simulink model "DC_motor_disc"  (R2022b)
settings: Solver=VariableStepAuto  StartTime=0.0  StopTime=1  RelTol=1e-7
PreLoadFcn:
  | P = eye(2);
  | Q_prev = [0.5 0; 0 0.5];
  | R_prev = eye(2);
PostLoadFcn:
  | P = eye(2);
  | Q_prev = [0.5 0; 0 0.5];
  | R_prev = eye(2);
InitFcn:
  | P = eye(2);
  | Q_prev = [0.5 0; 0 0.5];
  | R_prev = eye(2);
StartFcn:
  | P = eye(2);
  | Q_prev = [0.5 0; 0 0.5];
  | R_prev = eye(2);
values from neighbouring files (symbols this model uses):
  g = 9.81    [DC_motor_params.m]
  l = 0.05    [DC_motor_params.m]
  m = 5    [DC_motor_params.m]
  Ts = 10^-5    (= 1e-05)    [DC_motor_params.m]
undefined symbols (not defined in the file or in its folder): DiscIntNeverNeededParam, sigbuilder_block
libraries: simulink x3, spsControlledVoltageSourceLib x1, spsCurrentMeasurementLib x1, spsDCMachineLib x1, spsDCVoltageSourceLib x1, slpidlib x1, spsVoltageMeasurementLib x1, spspowerguiLib x1
settings Model: Creator=Pascal  LastModifiedBy=Pascal
settings DataIOCC: ReturnWorkspaceOutputs=off
settings DebuggingCC: AlgebraicLoopMsg=none
settings ModelReferenceCC: ModelReferenceMinAlgLoopOccurrences=on

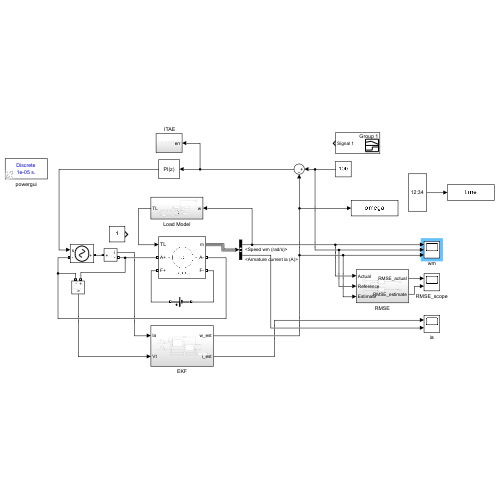
[thumbnail: Simulink's stored preview of the top-level diagram]
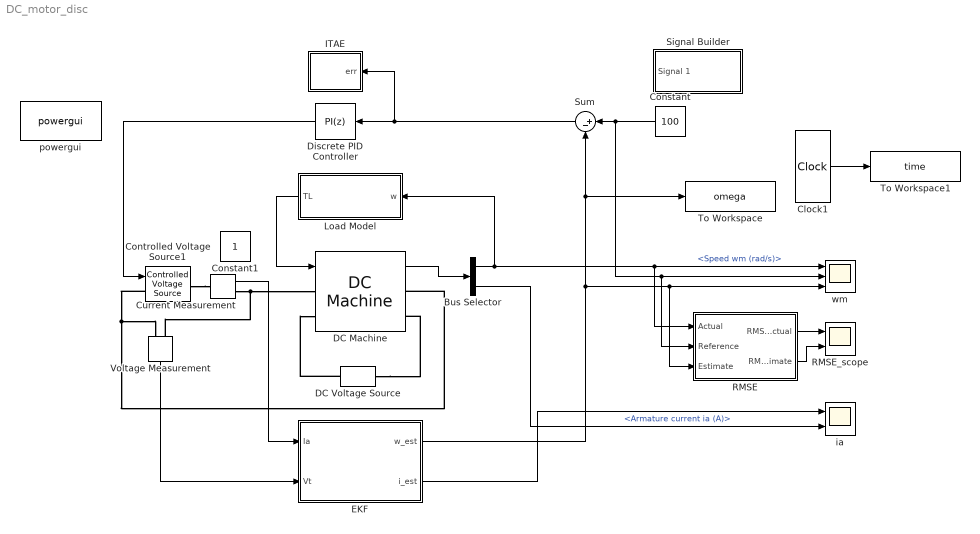
== system DC_motor_disc ==
  " ITAE" : Subsystem
  Bus Selector : BusSelector  OutputSignals=Speed wm (rad/s),Armature current ia (A)
  Clock1 : DigitalClock  SampleTime=Ts
  Constant : Constant  Value=100  SampleTime=Ts
  Constant1 : Constant
  Controlled Voltage Source1 : spsControlledVoltageSourceLib/Controlled Voltage Source  Initialize=off  Source_Type=DC  Amplitude=0  Phase=0  Frequency=0  Measurements=Voltage
  Current Measurement : spsCurrentMeasurementLib/Current Measurement  PhasorSimulation=off  OutputType=Complex  PSBequivalent=0
  DC Machine : spsDCMachineLib/DC Machine  PresetModel=No  MechanicalLoad=Torque TL  FieldType=Wound  ShowDetailedParameters=on  MeasurementBus=off  RLa=[2.581 0.028]  RLf=[240 120]  Laf=0.9483  MachineConstant=Torque constant (N.m/A)  Ke=1.8  Kt=1.8  J=0.02215  Bm=0.002953  Tf=0.5161  w0=0  Ifinit=1.25  TsPowergui=0  TsBlock=Ts
  DC Voltage Source : spsDCVoltageSourceLib/DC Voltage Source  Amplitude=300  Measurements=Voltage
  Discrete PID Controller : slpidlib/PID Controller  Controller=PI  Form=Parallel  TimeDomain=Discrete-time  UseExternalTs=off  SampleTime=-1  IntegratorMethod=Forward Euler  FilterMethod=Forward Euler  ControllerParametersSource=internal  P=1  I=20  UseKiTs=off  D=1  N=100  UseFilter=on  TunerSelectOption=Transfer Function Based (PID Tuner App)  InitialConditionSource=internal  InitialConditionForIntegrator=0  InitialConditionForFilter=0  DifferentiatorICPrevScaledInput=0  ExternalReset=none  TrackingMode=off  Kt=1  LimitOutput=off  SatLimitsSource=internal  UpperSaturationLimit=inf  LowerSaturationLimit=-inf  LinearizeAsGain=off  AntiWindupMode=none  Kb=1  LimitIntegrator=off  UpperIntegratorSaturationLimit=inf  LowerIntegratorSaturationLimit=-inf  POutMin=[]  POutMax=[]  IOutMin=[]  IOutMax=[]  DOutMin=[]  DOutMax=[]  NOutMin=[]  NOutMax=[]  SumOutMin=[]  SumOutMax=[]  SaturationOutMin=[]  SaturationOutMax=[]  PParamMin=[]  PParamMax=[]  IParamMin=[]  IParamMax=[]  DParamMin=[]  DParamMax=[]  NParamMin=[]  NParamMax=[]  KbParamMin=[]  KbParamMax=[]  KtParamMin=[]  KtParamMax=[]  KbOutMin=[]  KbOutMax=[]  KtOutMin=[]  KtOutMax=[]  IntegratorOutMin=[]  IntegratorOutMax=[]  FilterOutMin=[]  FilterOutMax=[]  SumI1OutMin=[]  SumI1OutMax=[]  SumI2OutMin=[]  SumI2OutMax=[]  SumI3OutMin=[]  SumI3OutMax=[]  SumI4OutMin=[]  SumI4OutMax=[]  SumDOutMin=[]  SumDOutMax=[]  DifferentiatorOutMin=[]  DifferentiatorOutMax=[]  FilterDiffOutCoefMin=[]  FilterDiffOutCoefMax=[]  ReciprocalOutMin=[]  ReciprocalOutMax=[]  SumDenOutMin=[]  SumDenOutMax=[]  SumNumOutMin=[]  SumNumOutMax=[]  DivideOutMin=[]  DivideOutMax=[]  UdiffTsProdOutMin=[]  UdiffTsProdOutMax=[]  NTsProdOutMin=[]  NTsProdOutMax=[]  UintegralTsProdOutMin=[]  UintegralTsProdOutMax=[]  UngainTsProdOutMin=[]  UngainTsProdOutMax=[]  ClampingZeroOutDataTypeStr=Inherit: Inherit via back propagation  ClampingZeroOutMin=[]  ClampingZeroOutMax=[]  FilterDenConstantOutDataTypeStr=Inherit: Inherit via back propagation  FilterDenConstantOutMin=[]  FilterDenConstantOutMax=[]  PCopyOutDataTypeStr=Inherit: Inherit via back propagation  PCopyOutMin=[]  PCopyOutMax=[]  NCopyOutDataTypeStr=Inherit: Inherit via back propagation  NCopyOutMin=[]  NCopyOutMax=[]  IntegratorContinuousStateAttributes=''  IntegratorStateMustResolveToSignalObject=off  IntegratorRTWStateStorageClass=Auto  FilterContinuousStateAttributes=''  FilterStateMustResolveToSignalObject=off  FilterRTWStateStorageClass=Auto  ParallelPVariant=InternalParameters  IdealPVariant=Disabled  IVariant=InternalParameters  DVariant=Disabled  IntegratorVariant=Discrete  SatVariant=Disabled  AWVariant=Passthrough  PCopyVariant=Disabled  TRVariant=Disabled  FdbkBlocksVariant=Forward  IdealPFdbkVariant=Disabled  SatFdbkVariant=Disabled  DerivativeFilterVariant=Disabled  NVariant=Disabled  NCopyVariant=Disabled_SignalSpec  FilterICVariant=Disabled  IntegratorICVariant=InternalICs  ExternalResetVariant=Disabled  TRSumVariant=Passthrough  SumFdbkVariant=Disabled  SumVariant=Sum_PI  TsampFilterVariant=InternalTs  TsampNgainVariant=Passthrough  TsampIntegralVariant=Passthrough  ExternalSaturationOutDataTypeStr=Inherit: Same as second input
      settings: LibrarySourceBlock=hdlsllib/Discrete/Discrete PID Controller
  EKF : Subsystem
  Load Model : Subsystem
  RMSE : Subsystem
  RMSE_scope : Scope  NumInputPorts=2
  Signal Builder : Subsystem  Tag=STV Subsys  LoadFcn=sigbuilder_block('load');  StartFcn=sigbuilder_block('start');  StopFcn=sigbuilder_block('stop');  ClipboardFcn=sigbuilder_block('clipboard');  mask(Sigbuilder block){tuvar=[0:10]}
      mask help: Simulink:masks:SigbuilderBlock_MD
      mask init:
      | if ~strcmp(get_param(bdroot(gcbh),'SimulationStatus'),'stopped') tuvar = sigbuilder_block('maskInit'); end
      settings: CopyFcn=sigbuilder_block('copy');  DeleteFcn=sigbuilder_block('delete');  ModelCloseFcn=sigbuilder_block('modelClose');  PreSaveFcn=sigbuilder_block('preSave');  PauseFcn=sigbuilder_block('pause');  ContinueFcn=sigbuilder_block('continue');  NameChangeFcn=sigbuilder_block('namechange');  OpenFcn=sigbuilder_block('open',[276 72 550.5 362.5 ]);  CloseFcn=sigbuilder_block('close');
      mask Display: plot(0, 0, 100, 100,[2, 2, 32, 32, 2], [68, 8, 8, 68, 68],[32, 2], [38, 38], [32, 19, 2],[53, 60, 44], [32, 17, 17, 2],[16, 16, 31, 31]);txt = getActiveGroup(gcbh);text(2, 100, txt,'verticalAlignment', 'top');
  Sum : Sum  Inputs=|+-
  To Workspace : ToWorkspace  VariableName=omega  SampleTime=-1
      settings: Save2DSignal=2-D array (concatenate along first dimension)
  To Workspace1 : ToWorkspace  VariableName=time  SampleTime=Ts
      settings: Save2DSignal=2-D array (concatenate along first dimension)
  Voltage Measurement : spsVoltageMeasurementLib/Voltage Measurement  PhasorSimulation=off  OutputType=Complex  PSBequivalent=0
  ia : Scope  NumInputPorts=2
  powergui : spspowerguiLib/powergui  Priority=1  SimulationMode=Discrete  SampleTime=10e-6  frequency=60  Iterations=50  frequencyindice=0  Pbase=100e6  ErrMax=1e-4  UnitsV=kV  UnitsW=MW  buscounter=0  FunctionMessages=off  echomessages=off  EnableUseOfTLC=off  CurrentSourceSwitches=off  DisableSnubberDevices=off  DisableRonSwitches=off  DisableVfSwitches=off  DisplayEquations=off  AutomaticDiscreteSolvers=off  SolverType=Tustin/Backward Euler (TBE)  Interpol=off  ExternalGateDelay=off  methode=off  Ts=100  x0status=blocks  SPID=on  SwTol=0  HookPort=off  NonlinearTolerance=1e-4  nMaxIteration=100  ContinueOnMaxIteration=off  RestoreLinks=warning  ResistiveCurrentMeasurement=off  Frange=[0:2:500]  Ylog=off  Xlog=on  ShowGrid=off  save=off  variable=ZData  structure=0  ZoomFFT=off  StartTime=0.0  cycles=1  DisplayStyle=1  fundamental=60  FreqAxis=off  MaxFrequency=1000  frequencyindicesteady=1  RmsSteady=1  display=off
  wm : Scope  NumInputPorts=3
  wires:
  DC Machine/1 -> Bus Selector/1
  Bus Selector/1 -> Load Model/1(w), RMSE/1(Actual), wm/1  "<Speed wm (rad/s)>"
  Clock1/1 -> To Workspace1/1
  Sum/1 -> Discrete PID Controller/1, " ITAE"/1(err)
  Current Measurement/1 -> EKF/1(Ia)
  Voltage Measurement/1 -> EKF/2(Vt)
  EKF/1(w_est) -> Sum/2, To Workspace/1, RMSE/3(Estimate), wm/3
  Discrete PID Controller/1 -> Controlled Voltage Source1/1
  EKF/2(i_est) -> ia/1
  Constant/1 -> RMSE/2(Reference), wm/2, Sum/1
  Bus Selector/2 -> ia/2  "<Armature current ia (A)>"
  RMSE/1(RMSE_actual) -> RMSE_scope/1
  RMSE/2(RMSE_estimate) -> RMSE_scope/2
  Load Model/1(TL) -> DC Machine/1
  connections:
  Current Measurement/RConn1 -- Voltage Measurement/LConn1 -- DC Machine/LConn1
  Controlled Voltage Source1/RConn1 -- Current Measurement/LConn1
  Controlled Voltage Source1/LConn1 -- Voltage Measurement/LConn2 -- DC Machine/RConn1
  DC Voltage Source/RConn1 -- DC Machine/LConn2
  DC Voltage Source/LConn1 -- DC Machine/RConn2

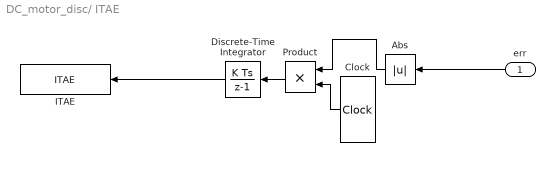
== system DC_motor_disc/ ITAE ==
  err : Inport
  Abs : Abs  SaturateOnIntegerOverflow=off
  Clock : DigitalClock  SampleTime=10e-06
  Discrete-Time Integrator : DiscreteIntegrator  SampleTime=-1  ICPrevOutput=DiscIntNeverNeededParam  ICPrevScaledInput=DiscIntNeverNeededParam
  ITAE : ToWorkspace  VariableName=ITAE  SampleTime=-1
      settings: Save2DSignal=2-D array (concatenate along first dimension)
  Product : Product
  wires:
  Clock/1 -> Product/2
  Product/1 -> Discrete-Time Integrator/1
  Discrete-Time Integrator/1 -> ITAE/1
  Abs/1 -> Product/1
  err/1 -> Abs/1

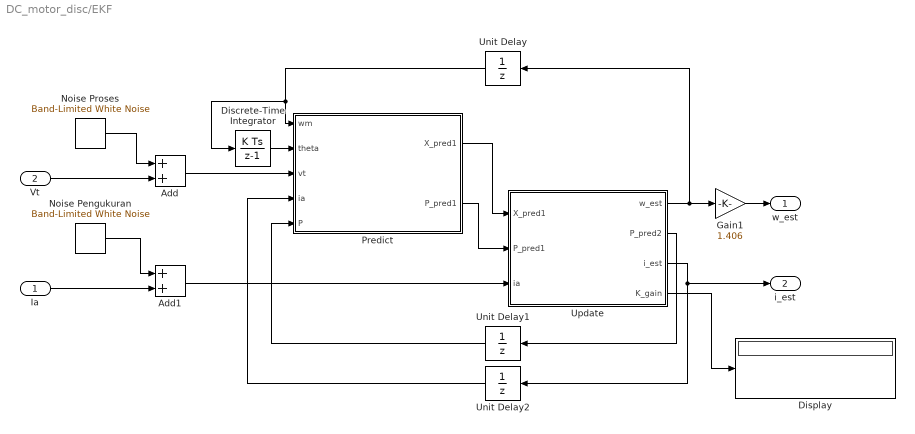
== system DC_motor_disc/EKF ==
  Ia : Inport
  Vt : Inport  Port=2
  Add : Sum
  Add1 : Sum
  Discrete-Time Integrator : DiscreteIntegrator  SampleTime=-1  ICPrevOutput=DiscIntNeverNeededParam  ICPrevScaledInput=DiscIntNeverNeededParam
  Display : Display
  Gain1 : Gain  Gain=1.406
  Noise Pengukuran : simulink/Sources/Band-Limited White Noise  Cov=[0.001]  Ts=0.1  seed=[23341]
  Noise Proses : simulink/Sources/Band-Limited White Noise  Cov=[0.1]  Ts=0.1  seed=[23341]
  Predict : MATLAB Function  TreatAsAtomicUnit=on
  Unit Delay : UnitDelay  SampleTime=-1  HasFrameUpgradeWarning=on
  Unit Delay1 : UnitDelay  SampleTime=-1  HasFrameUpgradeWarning=on
  Unit Delay2 : UnitDelay  SampleTime=-1  HasFrameUpgradeWarning=on
  Update : MATLAB Function  TreatAsAtomicUnit=on
  w_est : Outport  PortDimensions=1
  i_est : Outport  Port=2  PortDimensions=1
  wires:
  Discrete-Time Integrator/1 -> Predict/2(theta)
  Predict/1(X_pred1) -> Update/1(X_pred1)
  Predict/2(P_pred1) -> Update/2(P_pred1)
  Unit Delay/1 -> Discrete-Time Integrator/1, Predict/1(wm)
  Update/2(P_pred2) -> Unit Delay1/1
  Unit Delay1/1 -> Predict/5(P)
  Update/3(i_est) -> i_est/1, Unit Delay2/1
  Unit Delay2/1 -> Predict/4(ia)
  Add/1 -> Predict/3(vt)
  Vt/1 -> Add/2
  Ia/1 -> Add1/2
  Add1/1 -> Update/3(ia)
  Update/1(w_est) -> Gain1/1, Unit Delay/1
  Gain1/1 -> w_est/1
  Noise Proses/1 -> Add/1
  Noise Pengukuran/1 -> Add1/1
  Update/4(K_gain) -> Display/1

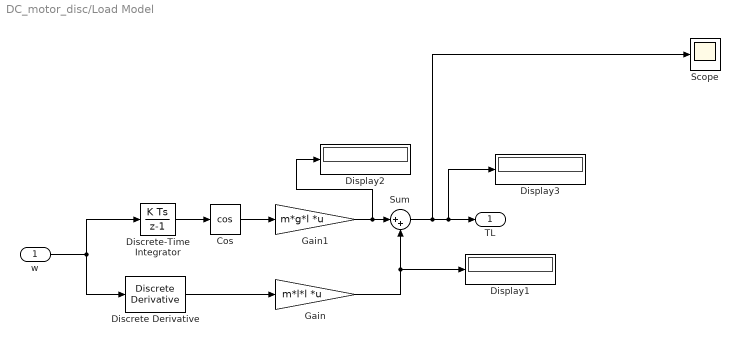
== system DC_motor_disc/Load Model ==
  w : Inport
  Cos : Trigonometry  Operator=cos
  Discrete Derivative : simulink/Discrete/Discrete Derivative  gainval=1.0  ICPrevScaledInput=0.0  OutMin=[]  OutMax=[]  OutDataType=fixdt(1, 16)  OutScaling=2^-10  DoSatur=off
  Discrete-Time Integrator : DiscreteIntegrator  SampleTime=-1  ICPrevOutput=DiscIntNeverNeededParam  ICPrevScaledInput=DiscIntNeverNeededParam
  Display1 : Display
  Display2 : Display
  Display3 : Display
  Gain : Gain  Gain=m*l*l  Multiplication=Matrix(K*u)
  Gain1 : Gain  Gain=m*g*l  Multiplication=Matrix(K*u)
  Scope : Scope
  Sum : Sum  Inputs=|++
  TL : Outport
  wires:
  w/1 -> Discrete-Time Integrator/1, Discrete Derivative/1
  Discrete-Time Integrator/1 -> Cos/1
  Discrete Derivative/1 -> Gain/1
  Cos/1 -> Gain1/1
  Gain/1 -> Display1/1, Sum/2
  Gain1/1 -> Display2/1, Sum/1
  Sum/1 -> Scope/1, Display3/1, TL/1

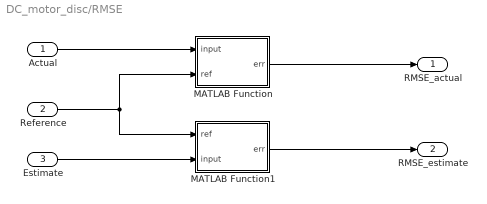
== system DC_motor_disc/RMSE ==
  Actual : Inport
  Reference : Inport  Port=2
  Estimate : Inport  Port=3
  MATLAB Function : MATLAB Function  TreatAsAtomicUnit=on
  MATLAB Function1 : MATLAB Function  TreatAsAtomicUnit=on
  RMSE_actual : Outport
  RMSE_estimate : Outport  Port=2
  wires:
  Estimate/1 -> MATLAB Function1/2(input)
  Actual/1 -> MATLAB Function/1(input)
  MATLAB Function1/1(err) -> RMSE_estimate/1
  Reference/1 -> MATLAB Function1/1(ref), MATLAB Function/2(ref)
  MATLAB Function/1(err) -> RMSE_actual/1

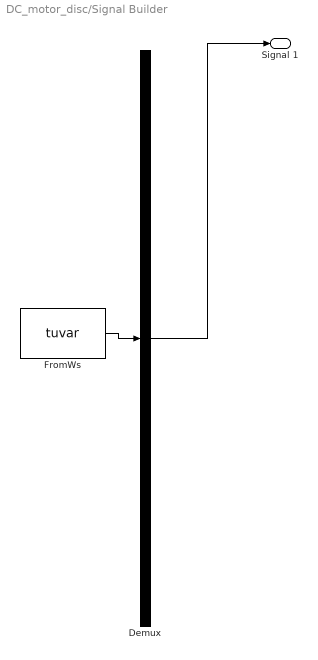
== system DC_motor_disc/Signal Builder ==
  Demux : Demux  Tag=STV Demux  Outputs=1
      settings: DisplayOption=none
  FromWs : FromWorkspace  Tag=STV FromWs  VariableName=tuvar
      SigBuilderData=|
      | common.afterFinalStr = 'Extrapolate'
      | common.sampleTime = 0
      | dataSet.timeRange = [0 3]
      | dataSet.name = 'Group 1'
      | sbobj.Groups.Name = 'Group 1'
      | sbobj.Groups.Signals.Name = 'Signal 1'
      | sbobj.Groups.Signals.XData = [0 1 1 2 3]
      | sbobj.Groups.Signals.YData = [100 100 50 50 20]
      | sbobj.Groups.TimeRange = [0 3]
  Signal 1 : Outport  Tag=STV Outport
  wires:
  FromWs/1 -> Demux/1
  Demux/1 -> Signal 1/1

== matlab function DC_motor_disc/EKF/Update ==
  data: w_est output; X_pred1 input; P_pred1 input; P_pred2 output; ia input; i_est output; K_gain output
function [w_est, P_pred2, i_est, K_gain] = fcn(X_pred1, P_pred1, ia)

Hk = [0 0;0 1]; % jacobian
R = [0.5 0; 0 0.5]; % kovarians proses

yk = Hk*[0;ia]; % vektor observasi
Sk = Hk*P_pred1*Hk' + R; % kovarians inovasi

K_gain = P_pred1*Hk'*(Sk^-1); % kalman gain

X_pred2 = X_pred1 + K_gain*(yk - Hk*X_pred1); % estimasi state
P_pred2 = P_pred1*(eye(2)-K_gain*Hk); % estimasi kovarians prediksi

w_est = X_pred2(1); % estimasi kecepatan
i_est = X_pred2(2); % estimasi arus

== matlab function DC_motor_disc/RMSE/MATLAB Function ==
  data: input input; ref input; err output
function err = mse(input, ref)

err = sqrt(immse(ref, input));

== matlab function DC_motor_disc/RMSE/MATLAB Function1 ==
  data: ref input; input input; err output
function err = mse(ref, input)

err = sqrt(immse(ref, input));

== matlab function DC_motor_disc/EKF/Predict ==
  data: X_pred1 output; P_pred1 output; wm input; theta input; vt input; ia input; P input
function [X_pred1, P_pred1] = fcn(wm,theta,vt,ia,P)

w_est = 1*wm + 0.0005*ia + (-7.0677e-04*cos(theta)-1.4873e-04);
i_est = -0.0006*wm + 0.9991*ia + 3.5714e-04*vt;
X_pred1 = [w_est; i_est]; % prediksi state

Fk= [1.0000 0.0005; % jacobian
    -0.0006 0.9991];
Q =[0.5 0; 0 0.5]; % kovarians proses

P_pred1 = Fk*P*Fk'+ Q; % kovarians prediksi
